simulink model "PIcontroller"  (R2019a)
settings: Solver=VariableStepAuto  StartTime=0.0  StopTime=60  RelTol=1e-3
values from neighbouring files (symbols this model uses):
  m = 20*log10(abs(K))    [butterworth.m]
undefined symbols (not defined in the file or in its folder): kf, v0
settings Model: Creator=user  LastModifiedBy=user

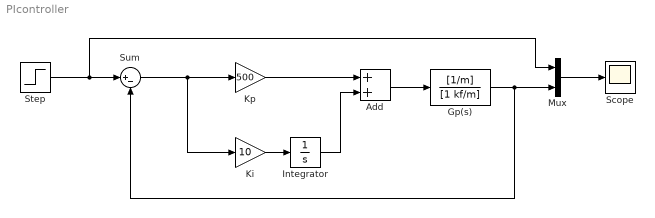
== system PIcontroller ==
  Add : Sum
  Gp(s) : TransferFcn  Numerator=[1/m]  Denominator=[1 kf/m]
  Integrator : Integrator
  Ki : Gain  Gain=10
  Kp : Gain  Gain=500
  Mux : Mux  Inputs=2
  Scope : Scope
  Step : Step  After=v0  SampleTime=0
  Sum : Sum  Inputs=|+-
  wires:
  Add/1 -> Gp(s)/1
  Kp/1 -> Add/1
  Integrator/1 -> Add/2
  Ki/1 -> Integrator/1
  Step/1 -> Mux/1, Sum/1
  Sum/1 -> Ki/1, Kp/1
  Gp(s)/1 -> Mux/2, Sum/2
  Mux/1 -> Scope/1
